simulink model "sampleModel306"  (R2021b)
settings: Solver=VariableStepAuto  StartTime=0.0  StopTime=10.0  RelTol=1e-3
undefined symbols (not defined in the file or in its folder): DiscIntNeverNeededParam
libraries: simulink x5, slpidlib x1
settings Model: Creator=user  LastModifiedBy=user

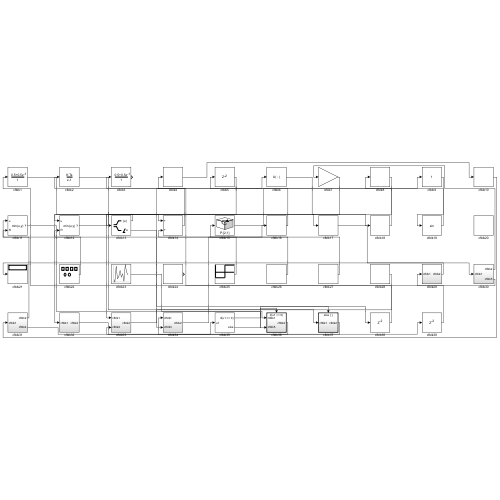
[thumbnail: Simulink's stored preview of the top-level diagram]
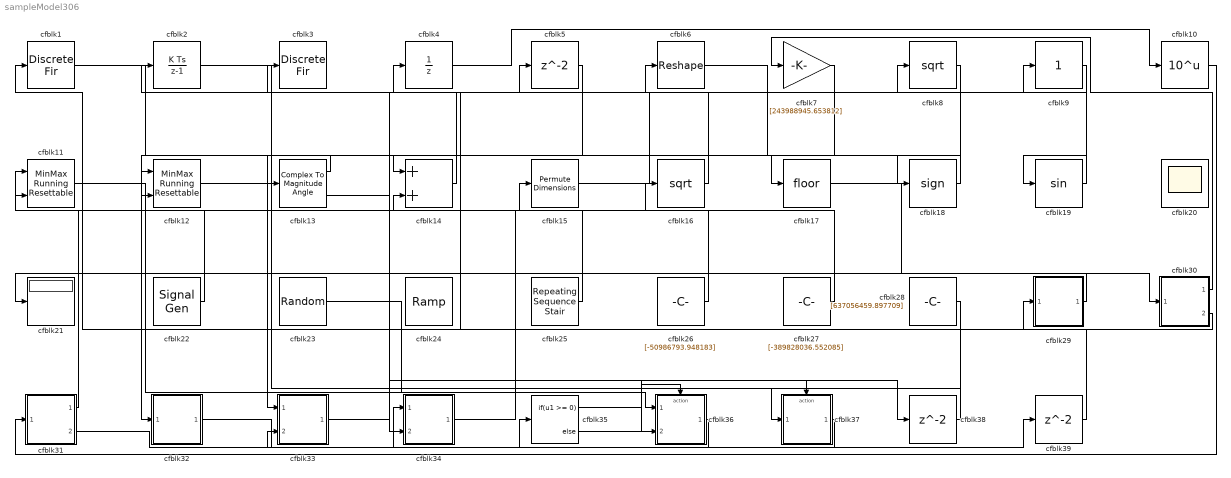
== system sampleModel306 ==
  cfblk1 : DiscreteFir  SampleTime=1
  cfblk10 : Math  Operator=10^u  SaturateOnIntegerOverflow=on
  cfblk11 : simulink/Math Operations/MinMax Running Resettable  Function=min  vinit=0.0
  cfblk12 : simulink/Math Operations/MinMax Running Resettable  Function=min  vinit=0.0
  cfblk13 : ComplexToMagnitudeAngle
  cfblk14 : Sum
  cfblk15 : PermuteDimensions
  cfblk16 : Sqrt  SaturateOnIntegerOverflow=on
  cfblk17 : Rounding
  cfblk18 : Signum
  cfblk19 : Trigonometry
  cfblk2 : DiscreteIntegrator  ICPrevOutput=DiscIntNeverNeededParam  ICPrevScaledInput=DiscIntNeverNeededParam
  cfblk20 : Scope
      settings: Floating=on
  cfblk21 : Display
  cfblk22 : SignalGenerator  WaveForm=square  Amplitude=[-45260389.677650]  Units=rad/sec
  cfblk23 : UniformRandomNumber  Minimum=[-9452381746.863241]  Maximum=[1946186997.231335]  Seed=[5289279.000000]  SampleTime=0.1
  cfblk24 : simulink/Sources/Ramp  slope=[-3910.090914]  start=[46.491464]  InitialOutput=[784005.839942]
  cfblk25 : simulink/Sources/Repeating Sequence Stair  OutValues=[-694649281.166414, 877497449.212925]  tsamp=-1  OutMin=[]  OutMax=[]  OutDataTypeStr=double  OutputDataTypeScalingMode=double  OutDataType=fixdt(0,8)  ConRadixGroup=Best Precision: Vector-wise  OutScaling=2^-12
  cfblk26 : Constant  Value=[-50986793.948183]  SampleTime=1
  cfblk27 : Constant  Value=[-389828036.552085]  SampleTime=1
  cfblk28 : Constant  Value=[637056459.897709]  SampleTime=1
  cfblk29 : Subsystem
  cfblk3 : DiscreteFir  SampleTime=1
  cfblk30 : Subsystem
  cfblk31 : Subsystem
  cfblk32 : Subsystem
  cfblk33 : Subsystem
  cfblk34 : Subsystem
  cfblk35 : If  IfExpression=u1 >= 0  SampleTime=1
  cfblk36 : Subsystem  TreatAsAtomicUnit=on
  cfblk37 : Subsystem  TreatAsAtomicUnit=on
  cfblk38 : Delay  SampleTime=1
  cfblk39 : Delay  SampleTime=1
  cfblk4 : UnitDelay  HasFrameUpgradeWarning=on
  cfblk5 : Delay  SampleTime=1
  cfblk6 : Reshape
  cfblk7 : Gain  Gain=[243988945.653812]
  cfblk8 : Sqrt  SaturateOnIntegerOverflow=on
  cfblk9 : simulink/Math Operations/Slider Gain  gain=1  low=0  high=2
  wires:
  cfblk12/1 -> cfblk14/1
  cfblk17/1 -> cfblk30/1(cfblk1)
  cfblk15/1 -> cfblk9/1
  cfblk11/1 -> cfblk36/1(cfblk1)
  cfblk27/1 -> cfblk14/2
  cfblk25/1 -> cfblk15/1
  cfblk1/1 -> cfblk17/1
  cfblk30/1(cfblk2) -> cfblk7/1
  cfblk37/1(cfblk2) -> cfblk34/1(cfblk1)
  cfblk14/1 -> cfblk2/1
  cfblk5/1 -> cfblk33/1(cfblk1)
  cfblk9/1 -> cfblk19/1
  cfblk32/1(cfblk2) -> cfblk35/1
  cfblk33/1(cfblk2) -> cfblk6/1
  cfblk2/1 -> cfblk37/1(cfblk1)
  cfblk8/1 -> cfblk32/1(cfblk1)
  cfblk31/1(cfblk2) -> cfblk11/1
  cfblk36/1(cfblk2) -> cfblk33/2(cfblk4)
  cfblk26/1 -> cfblk11/2
  cfblk10/1 -> cfblk31/1(cfblk1)
  cfblk13/1 -> cfblk12/1
  cfblk16/1 -> cfblk5/1
  cfblk34/1(cfblk2) -> cfblk16/1
  cfblk28/1 -> cfblk34/2(cfblk3)
  cfblk6/1 -> cfblk18/1
  cfblk7/1 -> cfblk13/1
  cfblk4/1 -> cfblk10/1
  cfblk19/1 -> cfblk8/1
  cfblk22/1 -> cfblk12/2
  cfblk29/1(cfblk2) -> cfblk21/1
  cfblk23/1 -> cfblk36/2(cfblk5)
  cfblk18/1 -> cfblk3/1
  cfblk30/2(cfblk5) -> cfblk29/1(cfblk1)
  cfblk35/1 -> cfblk36/Action
  cfblk35/2 -> cfblk37/Action
  cfblk13/2 -> cfblk38/1
  cfblk38/1 -> cfblk1/1
  cfblk31/2(cfblk4) -> cfblk39/1
  cfblk39/1 -> cfblk4/1

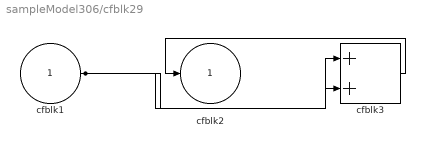
== system sampleModel306/cfblk29 ==
  cfblk1 : Inport
  cfblk3 : Sum
  cfblk2 : Outport
  wires:
  cfblk3/1 -> cfblk2/1
  cfblk1/1 -> cfblk3/1, cfblk3/2

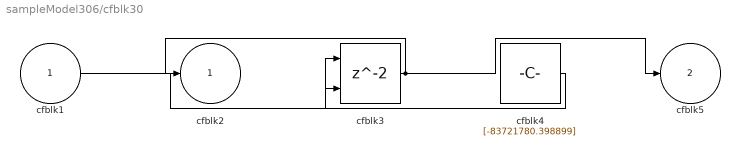
== system sampleModel306/cfblk30 ==
  cfblk1 : Inport
  cfblk3 : Delay  ShowEnablePort=on  SampleTime=1
      settings: InputPortMap=u0,e6
  cfblk4 : Constant  Value=[-83721780.398899]  SampleTime=1
  cfblk2 : Outport
  cfblk5 : Outport  Port=2
  wires:
  cfblk3/1 -> cfblk5/1, cfblk2/1
  cfblk4/1 -> cfblk3/1
  cfblk1/1 -> cfblk3/2

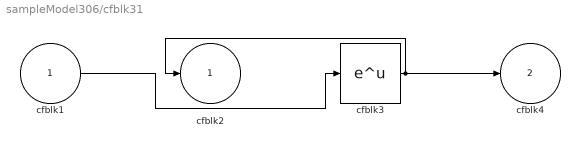
== system sampleModel306/cfblk31 ==
  cfblk1 : Inport
  cfblk3 : Math  SaturateOnIntegerOverflow=on
  cfblk2 : Outport
  cfblk4 : Outport  Port=2
  wires:
  cfblk3/1 -> cfblk2/1, cfblk4/1
  cfblk1/1 -> cfblk3/1

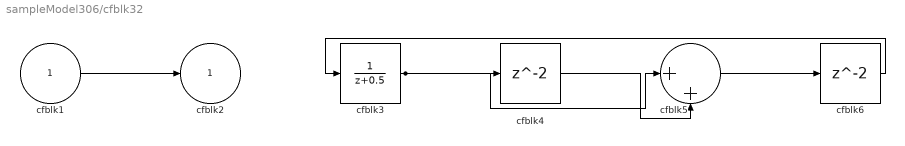
== system sampleModel306/cfblk32 ==
  cfblk1 : Inport
  cfblk3 : DiscreteTransferFcn  SampleTime=1
  cfblk4 : Delay  SampleTime=1
  cfblk5 : Sum  Inputs=|++
  cfblk6 : Delay  SampleTime=1
  cfblk2 : Outport
  wires:
  cfblk1/1 -> cfblk2/1
  cfblk3/1 -> cfblk5/1, cfblk4/1
  cfblk4/1 -> cfblk5/2
  cfblk5/1 -> cfblk6/1
  cfblk6/1 -> cfblk3/1

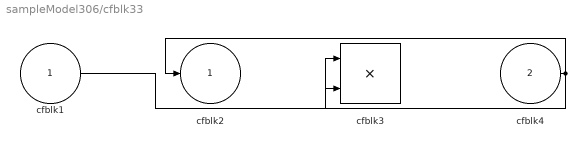
== system sampleModel306/cfblk33 ==
  cfblk1 : Inport
  cfblk4 : Inport  Port=2
  cfblk3 : Product
  cfblk2 : Outport
  wires:
  cfblk4/1 -> cfblk2/1, cfblk3/2
  cfblk1/1 -> cfblk3/1

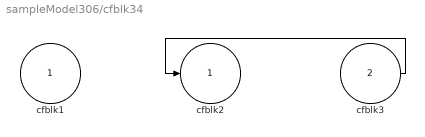
== system sampleModel306/cfblk34 ==
  cfblk1 : Inport
  cfblk3 : Inport  Port=2
  cfblk2 : Outport
  wires:
  cfblk3/1 -> cfblk2/1

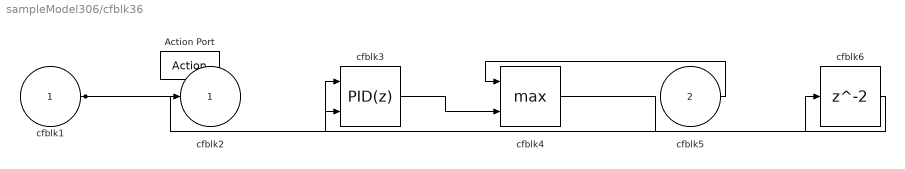
== system sampleModel306/cfblk36 ==
  cfblk1 : Inport
  cfblk5 : Inport  Port=2
  Action Port : ActionPort  ActionPortLabel=if(u1 >= 0)
  cfblk3 : slpidlib/PID Controller (2DOF)  Controller=PID  Form=Parallel  TimeDomain=Discrete-time  UseExternalTs=off  SampleTime=-1  IntegratorMethod=Forward Euler  FilterMethod=Forward Euler  ControllerParametersSource=internal  P=1  I=1  D=0  UseFilter=on  N=100  b=1  c=1  TunerSelectOption=Transfer Function Based (PID Tuner App)  InitialConditionSource=internal  InitialConditionForIntegrator=0  InitialConditionForFilter=0  DifferentiatorICPrevScaledInput=0  ExternalReset=none  TrackingMode=off  Kt=1  LimitOutput=off  SatLimitsSource=internal  UpperSaturationLimit=inf  LowerSaturationLimit=-inf  LinearizeAsGain=off  AntiWindupMode=none  Kb=1  POutMin=[]  POutMax=[]  IOutMin=[]  IOutMax=[]  DOutMin=[]  DOutMax=[]  NOutMin=[]  NOutMax=[]  bOutMin=[]  bOutMax=[]  cOutMin=[]  cOutMax=[]  SumOutMin=[]  SumOutMax=[]  SaturationOutMin=[]  SaturationOutMax=[]  PParamMin=[]  PParamMax=[]  IParamMin=[]  IParamMax=[]  DParamMin=[]  DParamMax=[]  NParamMin=[]  NParamMax=[]  bParamMin=[]  bParamMax=[]  cParamMin=[]  cParamMax=[]  KbParamMin=[]  KbParamMax=[]  KtParamMin=[]  KtParamMax=[]  KbOutMin=[]  KbOutMax=[]  KtOutMin=[]  KtOutMax=[]  IntegratorOutMin=[]  IntegratorOutMax=[]  FilterOutMin=[]  FilterOutMax=[]  SumI1OutMin=[]  SumI1OutMax=[]  SumI2OutMin=[]  SumI2OutMax=[]  SumI3OutMin=[]  SumI3OutMax=[]  SumI4OutMin=[]  SumI4OutMax=[]  SumDOutMin=[]  SumDOutMax=[]  Sum1OutMin=[]  Sum1OutMax=[]  Sum2OutMin=[]  Sum2OutMax=[]  Sum3OutMin=[]  Sum3OutMax=[]  DifferentiatorOutMin=[]  DifferentiatorOutMax=[]  FilterDiffOutCoefMin=[]  FilterDiffOutCoefMax=[]  ReciprocalOutMin=[]  ReciprocalOutMax=[]  SumDenOutMin=[]  SumDenOutMax=[]  SumNumOutMin=[]  SumNumOutMax=[]  DivideOutMin=[]  DivideOutMax=[]  UdiffTsProdOutMin=[]  UdiffTsProdOutMax=[]  NTsProdOutMin=[]  NTsProdOutMax=[]  UintegralTsProdOutMin=[]  UintegralTsProdOutMax=[]  UngainTsProdOutMin=[]  UngainTsProdOutMax=[]  IntegratorContinuousStateAttributes=''  IntegratorStateMustResolveToSignalObject=off  IntegratorRTWStateStorageClass=Auto  FilterContinuousStateAttributes=''  FilterStateMustResolveToSignalObject=off  FilterRTWStateStorageClass=Auto  ParallelPVariant=InternalParameters  IdealPVariant=Disabled  IVariant=InternalParameters  DVariant=InternalParameters  bVariant=InternalParameters  cVariant=InternalParameters  IntegratorVariant=Discrete  SatVariant=Disabled  AWVariant=Passthrough  PCopyVariant=Disabled  TRVariant=Disabled  FdbkBlocksVariant=Forward  IdealPFdbkVariant=Disabled  SatFdbkVariant=Disabled  DerivativeFilterVariant=ForwardEulerFilter  NVariant=InternalParameters  NCopyVariant=Disabled  FilterICVariant=InternalICsFilter  IntegratorICVariant=InternalICs  ExternalResetVariant=Disabled  TRSumVariant=Passthrough  SumFdbkVariant=Disabled  SumVariant=Sum_PID  TsampFilterVariant=InternalTs  TsampNgainVariant=Passthrough  TsampIntegralVariant=Passthrough  ExternalSaturationOutDataTypeStr=Inherit: Same as second input
      settings: SourceProductBaseCode=SL
  cfblk4 : MinMax  Function=max  Inputs=2
  cfblk6 : Delay
  cfblk2 : Outport
  wires:
  cfblk1/1 -> cfblk3/1, cfblk2/1
  cfblk5/1 -> cfblk4/1
  cfblk3/1 -> cfblk4/2
  cfblk4/1 -> cfblk6/1
  cfblk6/1 -> cfblk3/2

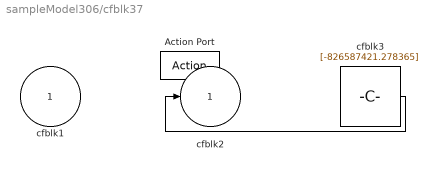
== system sampleModel306/cfblk37 ==
  cfblk1 : Inport
  Action Port : ActionPort  ActionPortLabel=else
  cfblk3 : Constant  Value=[-826587421.278365]  SampleTime=1
  cfblk2 : Outport
  wires:
  cfblk3/1 -> cfblk2/1
